simulink model "Vehicle_Model_14DOF"  (R2020a)
settings: Solver=ode23s  StartTime=0.0  StopTime=8  RelTol=1e-2  EnableMultiTasking=on
model workspace (MAT data in the model file):
  Csfl = 100
  Csfr = 100
  Csrl = 100
  Csrr = 100
  Hp = 0.35
  Ksfl = 100
  Ksfr = 100
  Ksrl = 100
  Ksrr = 100
undefined symbols (not defined in the file): sigbuilder_block
libraries: simulink_extras x6, simulink x1
(part 2 of 3)

== system Vehicle_Model_14DOF/Full vehicle 14 D.O.F /Vehicle Handling model 7D.O.F /Lateral Axis D.o.f  ==
  "ackerman outer " : Inport
  "ackerman in " : Inport  Port=2
  Fyfl : Inport  Port=3
  Fyrr : Inport  Port=4
  Fxfl : Inport  Port=5
  Fxfr : Inport  Port=6
  Fyfr : Inport  Port=7
  Fyrl : Inport  Port=8
  Vx : Inport  Port=9
  "Yaw rate " : Inport  Port=10
  "Centripital force deduction ay " : MATLAB Function  TreatAsAtomicUnit=on
  Gain : Gain  Gain=1/Ms
  Integrator : Integrator
  Integrator2 : Integrator
  MATLAB Function : MATLAB Function  TreatAsAtomicUnit=on
  Scope : Scope  NumInputPorts=2
  Scope1 : Scope
  product : Product  Inputs=**
  Y : Outport  VectorParamsAs1DForOutWhenUnconnected=off
  ay : Outport  Port=2  VectorParamsAs1DForOutWhenUnconnected=off
  Vy : Outport  Port=3  VectorParamsAs1DForOutWhenUnconnected=off
  Ay load transfer : Outport  Port=4
  wires:
  MATLAB Function/1(AY) -> Scope1/1, Gain/1  "Sprung accelration"
  Integrator2/1 -> Y/1
  Integrator/1 -> Integrator2/1, Vy/1
  "Centripital force deduction ay "/1(ay) -> ay/1, Integrator/1
  Gain/1 -> Ay load transfer/1, Scope/1, "Centripital force deduction ay "/1(Vy_dot)  "Ay"
  Vx/1 -> product/2, "Centripital force deduction ay "/2(Vx)
  "Yaw rate "/1 -> product/1, "Centripital force deduction ay "/3(Yr)
  "ackerman outer "/1 -> MATLAB Function/1(A_o)
  Fyfl/1 -> MATLAB Function/3(Fyfl)
  Fxfl/1 -> MATLAB Function/4(Fxfl)
  Fyfr/1 -> MATLAB Function/5(Fyfr)
  Fxfr/1 -> MATLAB Function/6(Fxfr)
  Fyrl/1 -> MATLAB Function/7(Fyrl)
  Fyrr/1 -> MATLAB Function/8(Fyrr)
  "ackerman in "/1 -> MATLAB Function/2(A_i)
  product/1 -> Scope/2  "V R"

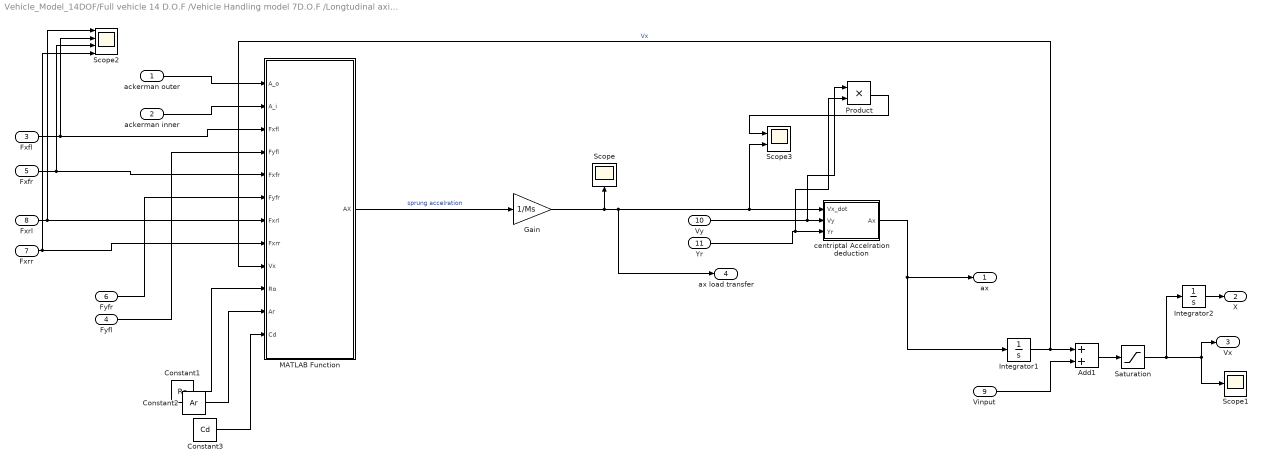
== system Vehicle_Model_14DOF/Full vehicle 14 D.O.F /Vehicle Handling model 7D.O.F /Longtudinal axis D.O.F  ==
  ackerman outer : Inport
  ackerman inner : Inport  Port=2
  Fxfl : Inport  Port=3
  Fyfl : Inport  Port=4
  Fxfr : Inport  Port=5
  Fyfr : Inport  Port=6
  Fxrr : Inport  Port=7
  Fxrl : Inport  Port=8
  Vinput : Inport  Port=9
  "Vy " : Inport  Port=10
  "Yr " : Inport  Port=11
  Add1 : Sum
  Constant1 : Constant  Value=Ro
  Constant2 : Constant  Value=Ar
  Constant3 : Constant  Value=Cd
  Gain : Gain  Gain=1/Ms
  Integrator1 : Integrator
  Integrator2 : Integrator
  MATLAB Function : MATLAB Function  TreatAsAtomicUnit=on
  Product : Product
  Saturation : Saturate  UpperLimit=inf  LowerLimit=0
  Scope : Scope
  Scope1 : Scope
  Scope2 : Scope  NumInputPorts=4
  Scope3 : Scope  NumInputPorts=2
  "centriptal Accelration deduction " : MATLAB Function  TreatAsAtomicUnit=on
  "ax " : Outport  VectorParamsAs1DForOutWhenUnconnected=off
  X : Outport  Port=2  VectorParamsAs1DForOutWhenUnconnected=off
  Vx : Outport  Port=3  VectorParamsAs1DForOutWhenUnconnected=off
  ax load transfer : Outport  Port=4
  wires:
  MATLAB Function/1(AX) -> Gain/1  "sprung accelration"
  Add1/1 -> Saturation/1
  Integrator2/1 -> X/1
  Gain/1 -> ax load transfer/1, "centriptal Accelration deduction "/1(Vx_dot), Scope3/2, Scope/1
  Vinput/1 -> Add1/2
  "centriptal Accelration deduction "/1(Ax) -> Integrator1/1, "ax "/1
  Integrator1/1 -> MATLAB Function/9(Vx), Add1/1  "Vx"
  "Yr "/1 -> Product/2, "centriptal Accelration deduction "/3(Yr)
  "Vy "/1 -> Product/1, "centriptal Accelration deduction "/2(Vy)
  ackerman outer/1 -> MATLAB Function/1(A_o)
  Fxfl/1 -> Scope2/2, MATLAB Function/3(Fxfl)
  Fyfl/1 -> MATLAB Function/4(Fyfl)
  Fxfr/1 -> Scope2/3, MATLAB Function/5(Fxfr)
  Fyfr/1 -> MATLAB Function/6(Fyfr)
  Fxrl/1 -> Scope2/1, MATLAB Function/7(Fxrl)
  Fxrr/1 -> Scope2/4, MATLAB Function/8(Fxrr)
  ackerman inner/1 -> MATLAB Function/2(A_i)
  Constant1/1 -> MATLAB Function/10(Ro)
  Constant2/1 -> MATLAB Function/11(Ar)
  Constant3/1 -> MATLAB Function/12(Cd)
  Saturation/1 -> Integrator2/1, Vx/1, Scope1/1
  Product/1 -> Scope3/1

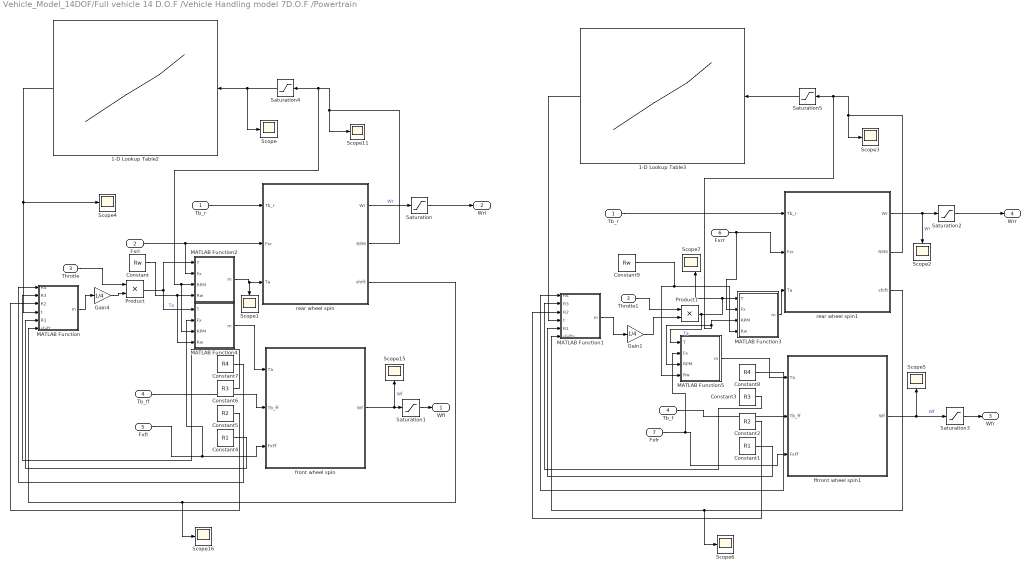
== system Vehicle_Model_14DOF/Full vehicle 14 D.O.F /Vehicle Handling model 7D.O.F /Powertrain  ==
  Tb_r : Inport
  Fxrl : Inport  Port=2
  Throtle : Inport  Port=3
  Tb_ff : Inport  Port=4
  "Fxfl " : Inport  Port=5
  Fxrr : Inport  Port=6
  Fxfr : Inport  Port=7
  1-D Lookup Table2 : Lookup_n-D  NumberOfTableDimensions=1  BreakpointsForDimension1=|  BreakpointsForDimension1FirstPoint=0  BreakpointsForDimension1Spacing=10000  Table=|  InternalRulePriority=Speed  RndMeth=Simplest  InputSameDT=on
      BreakpointsForDimension1=|
      | [ 999.991
      | 1500
      | 2000
      | 2500
      | 3000
      | 3500.01
      | 4000.02
      | 4500.01
      | 5000
      | 5500
      | 5999.99
      | 6500
      | 7000
      | 7500
      | 7999.99
      | 8499.99
      | 9000
      | 9500
      | 10000
      |   ]
      Table=|
      | [ 19.6089
      | 22.3386
      | 29.0552
      | 34.7654
      | 35.9299
      | 38.8977
      | 40.7484
      | 40.3784
      | 39.5416
      | 37.9236
      | 36.7992
      |  35.555
      | 
      | 34.3787
      | 33.134
      | 32.6401
      | 31.4746
      | 30.2131
      | 29.2355
      | 28.2404
      | ]
  1-D Lookup Table3 : Lookup_n-D  NumberOfTableDimensions=1  BreakpointsForDimension1=|  BreakpointsForDimension1FirstPoint=0  BreakpointsForDimension1Spacing=10000  Table=|  InternalRulePriority=Speed  RndMeth=Simplest  InputSameDT=on
      BreakpointsForDimension1=|
      | [ 999.991
      | 1500
      | 2000
      | 2500
      | 3000
      | 3500.01
      | 4000.02
      | 4500.01
      | 5000
      | 5500
      | 5999.99
      | 6500
      | 7000
      | 7500
      | 7999.99
      | 8499.99
      | 9000
      | 9500
      | 10000
      |   ]
      Table=|
      | [ 19.6089
      | 22.3386
      | 29.0552
      | 34.7654
      | 35.9299
      | 38.8977
      | 40.7484
      | 40.3784
      | 39.5416
      | 37.9236
      | 36.7992
      |  35.555
      | 
      | 34.3787
      | 33.134
      | 32.6401
      | 31.4746
      | 30.2131
      | 29.2355
      | 28.2404
      | ]
  Constant : Constant  Value=Rw
  Constant1 : Constant  Value=R1
  Constant2 : Constant  Value=R2
  Constant3 : Constant  Value=R3
  Constant4 : Constant  Value=R1
  Constant5 : Constant  Value=R2
  Constant6 : Constant  Value=R3
  Constant7 : Constant  Value=R4
  Constant8 : Constant  Value=R4
  Constant9 : Constant  Value=Rw
  Gain1 : Gain  Gain=1/4
  Gain4 : Gain  Gain=1/4
  MATLAB Function : MATLAB Function  TreatAsAtomicUnit=on
  MATLAB Function1 : MATLAB Function  TreatAsAtomicUnit=on
  MATLAB Function2 : MATLAB Function  TreatAsAtomicUnit=on
  MATLAB Function3 : MATLAB Function  TreatAsAtomicUnit=on
  MATLAB Function4 : MATLAB Function  TreatAsAtomicUnit=on
  MATLAB Function5 : MATLAB Function  TreatAsAtomicUnit=on
  Product : Product
  Product1 : Product
  Saturation{,1..3} (4 alike) : Saturate  UpperLimit=inf  LowerLimit=0.3745318
  Saturation4 : Saturate  UpperLimit=15000  LowerLimit=0
  Saturation5 : Saturate  UpperLimit=15000  LowerLimit=0
  Scope{,1..6,11,15..16} (10 alike) : Scope
  Scope7 : Scope  NumInputPorts=2
  "Tb_f " : InportShadow  Port=4
  "Tb_r " : InportShadow
  Throtle1 : InportShadow  Port=3
  ffrront wheel spin1 : Subsystem
  front wheel spin : Subsystem
  rear wheel spin : Subsystem
  rear wheel spin1 : Subsystem
  Wfl : Outport  VectorParamsAs1DForOutWhenUnconnected=off
  Wrl : Outport  Port=2  VectorParamsAs1DForOutWhenUnconnected=off
  Wfr : Outport  Port=3  VectorParamsAs1DForOutWhenUnconnected=off
  Wrr : Outport  Port=4  VectorParamsAs1DForOutWhenUnconnected=off
  wires:
  Fxrl/1 -> rear wheel spin/2(Fxr), MATLAB Function2/2(Fx)
  "Fxfl "/1 -> MATLAB Function4/2(Fx), front wheel spin/3(FxFf)
  1-D Lookup Table2/1 -> Scope4/1, MATLAB Function/4(t)
  rear wheel spin/2(RPM) -> MATLAB Function4/3(RPM), MATLAB Function2/3(RPM), Saturation4/1, Scope11/1
  MATLAB Function/1(m) -> Gain4/1
  rear wheel spin/1("Wr ") -> Saturation/1  "Wr"
  Tb_r/1 -> rear wheel spin/1(Tb_r)
  front wheel spin/1(Wf) -> Scope15/1, Saturation1/1  "Wf"
  Tb_ff/1 -> front wheel spin/2(Tb_ff)
  Gain4/1 -> Product/2
  rear wheel spin/3(shift) -> Scope16/1, MATLAB Function/6(shift)
  Constant4/1 -> MATLAB Function/5(R1)
  Constant5/1 -> MATLAB Function/3(R2)
  Throtle/1 -> Product/1
  Constant7/1 -> MATLAB Function/1(R4)
  Constant6/1 -> MATLAB Function/2(R3)
  Fxrr/1 -> MATLAB Function3/2(Fx), rear wheel spin1/2(Fxr)
  Fxfr/1 -> MATLAB Function5/2(Fx), ffrront wheel spin1/3(FxFf)
  1-D Lookup Table3/1 -> MATLAB Function1/4(t)
  rear wheel spin1/2(RPM) -> MATLAB Function5/3(RPM), MATLAB Function3/3(RPM), Saturation5/1, Scope3/1
  MATLAB Function1/1(m) -> Gain1/1
  rear wheel spin1/1("Wr ") -> Scope2/1, Saturation2/1  "Wr"
  Product1/1 -> MATLAB Function5/1(T), Scope7/2, MATLAB Function3/1(T)  "Ta"
  "Tb_r "/1 -> rear wheel spin1/1(Tb_r)
  ffrront wheel spin1/1(Wf) -> Scope5/1, Saturation3/1  "Wf"
  "Tb_f "/1 -> ffrront wheel spin1/2(Tb_ff)
  Gain1/1 -> Product1/2
  rear wheel spin1/3(shift) -> MATLAB Function1/6(shifts), Scope6/1
  Constant1/1 -> MATLAB Function1/5(R1)
  Constant2/1 -> MATLAB Function1/3(R2)
  Constant8/1 -> MATLAB Function1/1(R4)
  Constant3/1 -> MATLAB Function1/2(R3)
  Throtle1/1 -> Product1/1
  Saturation/1 -> Wrl/1
  Saturation1/1 -> Wfl/1
  Saturation2/1 -> Wrr/1
  Saturation3/1 -> Wfr/1
  Saturation4/1 -> 1-D Lookup Table2/1, Scope/1
  Saturation5/1 -> 1-D Lookup Table3/1
  Product/1 -> MATLAB Function4/1(T), MATLAB Function2/1(T)  "Ta"
  MATLAB Function2/1(m) -> Scope1/1, rear wheel spin/3(Ta)
  MATLAB Function3/1(m) -> rear wheel spin1/3(Ta)
  MATLAB Function4/1(m) -> front wheel spin/1(Ta)
  MATLAB Function5/1(m) -> ffrront wheel spin1/1(Ta)
  Constant/1 -> MATLAB Function4/4(Rw), MATLAB Function2/4(Rw)
  Constant9/1 -> MATLAB Function3/4(Rw), MATLAB Function5/4(Rw)

== system Vehicle_Model_14DOF/Full vehicle 14 D.O.F /Vehicle Handling model 7D.O.F /Slip angle and beta  ==
  ackerman angle outer : Inport
  "ackerman angle Inner " : Inport  Port=2
  Yaw rate : Inport  Port=3
  Vx : Inport  Port=4
  "Vy  " : Inport  Port=5
  Slip angle front : Subsystem
  Slip angle front1 : Subsystem
  Slip angle rear : Subsystem
  Slip angle rear1 : Subsystem
  "Vx  " : InportShadow  Port=4
  "Vx        " : InportShadow  Port=4
  "Vx         " : InportShadow  Port=4
  "Vy     " : InportShadow  Port=5
  "Vy        " : InportShadow  Port=5
  "Vy         " : InportShadow  Port=5
  "Yaw rate      " : InportShadow  Port=3
  "Yaw rate         " : InportShadow  Port=3
  "Yaw rate          " : InportShadow  Port=3
  alpha_fl : Outport  VectorParamsAs1DForOutWhenUnconnected=off
  alpha_fr : Outport  Port=2  VectorParamsAs1DForOutWhenUnconnected=off
  alpha_rl : Outport  Port=3  VectorParamsAs1DForOutWhenUnconnected=off
  alpha_rr : Outport  Port=4  VectorParamsAs1DForOutWhenUnconnected=off
  wires:
  Slip angle rear/1(alpha_R) -> alpha_rl/1  "rl"
  Slip angle front1/1(alpha_F) -> alpha_fr/1  "fl"
  Slip angle rear1/1(alpha_R) -> alpha_rr/1  "rl"
  ackerman angle outer/1 -> Slip angle front/2(Delta)
  "Vy     "/1 -> Slip angle front/3(Ydot)
  Yaw rate/1 -> Slip angle front/4(Psidot)
  Vx/1 -> Slip angle front/1(Xdot)
  "Vx        "/1 -> Slip angle front1/1(Xdot)
  "Yaw rate         "/1 -> Slip angle front1/4(Psidot)
  "Vy        "/1 -> Slip angle front1/3(Ydot)
  "ackerman angle Inner "/1 -> Slip angle front1/2(Delta)
  Slip angle front/1(alpha_F) -> alpha_fl/1  "fl"
  "Vy         "/1 -> Slip angle rear1/2(Ydot)
  "Yaw rate          "/1 -> Slip angle rear1/3(Psidot)
  "Vx         "/1 -> Slip angle rear1/1(Xdot)
  "Vy  "/1 -> Slip angle rear/2(Ydot)
  "Vx  "/1 -> Slip angle rear/1(Xdot)
  "Yaw rate      "/1 -> Slip angle rear/3(Psidot)

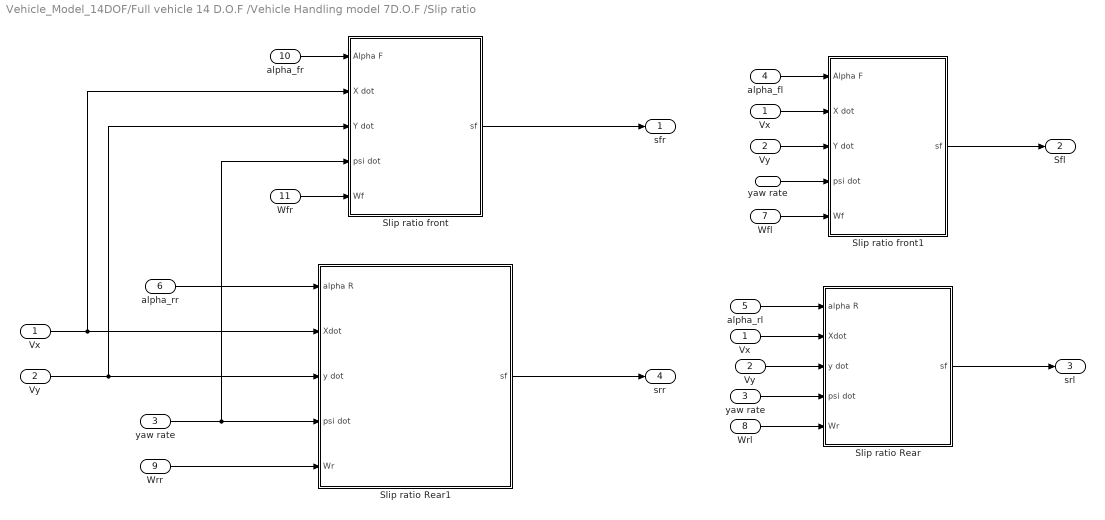
== system Vehicle_Model_14DOF/Full vehicle 14 D.O.F /Vehicle Handling model 7D.O.F /Slip ratio  ==
  "Vx " : Inport
  Vy : Inport  Port=2
  yaw rate : Inport  Port=3
  alpha_fl : Inport  Port=4
  "alpha_rl " : Inport  Port=5
  alpha_rr : Inport  Port=6
  "Wfl " : Inport  Port=7
  Wrl : Inport  Port=8
  Wrr : Inport  Port=9
  alpha_fr : Inport  Port=10
  Wfr : Inport  Port=11
  Slip ratio Rear : Subsystem
  Slip ratio Rear1 : Subsystem
  Slip ratio front : Subsystem
  Slip ratio front1 : Subsystem
  "Vx " : InportShadow
  "Vx " : InportShadow
  "Vy " : InportShadow  Port=2
  "Vy " : InportShadow  Port=2
  "yaw rate " : InportShadow  Port=3
  "yaw rate        " : InportShadow  Port=3
  sfr : Outport  VectorParamsAs1DForOutWhenUnconnected=off
  Sfl : Outport  Port=2  VectorParamsAs1DForOutWhenUnconnected=off
  srl : Outport  Port=3  VectorParamsAs1DForOutWhenUnconnected=off
  srr : Outport  Port=4  VectorParamsAs1DForOutWhenUnconnected=off
  wires:
  "yaw rate        "/1 -> Slip ratio front/4(psi dot), Slip ratio Rear1/4(psi dot)
  alpha_rr/1 -> Slip ratio Rear1/1(alpha R)
  "Vx "/1 -> Slip ratio front1/2(X dot)
  Vy/1 -> Slip ratio front1/3(Y dot)
  yaw rate/1 -> Slip ratio front1/4(psi dot)
  alpha_fl/1 -> Slip ratio front1/1(Alpha F)
  "Vx "/1 -> Slip ratio Rear/2(Xdot)
  "Vy "/1 -> Slip ratio Rear/3(y dot)
  "yaw rate "/1 -> Slip ratio Rear/4(psi dot)
  "alpha_rl "/1 -> Slip ratio Rear/1(alpha R)
  Wrr/1 -> Slip ratio Rear1/5(Wr)
  Wrl/1 -> Slip ratio Rear/5(Wr)
  "Wfl "/1 -> Slip ratio front1/5(Wf)
  Slip ratio Rear1/1(sf) -> srr/1
  Slip ratio front1/1(sf) -> Sfl/1
  Slip ratio Rear/1(sf) -> srl/1
  Slip ratio front/1(sf) -> sfr/1
  Wfr/1 -> Slip ratio front/5(Wf)
  alpha_fr/1 -> Slip ratio front/1(Alpha F)
  "Vy "/1 -> Slip ratio front/3(Y dot), Slip ratio Rear1/3(y dot)
  "Vx "/1 -> Slip ratio front/2(X dot), Slip ratio Rear1/2(Xdot)

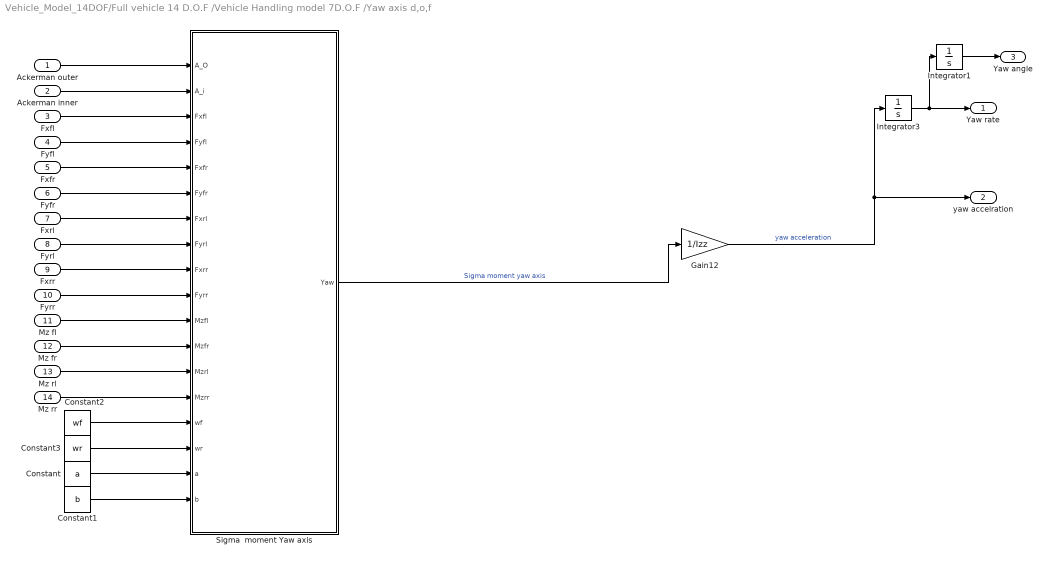
== system Vehicle_Model_14DOF/Full vehicle 14 D.O.F /Vehicle Handling model 7D.O.F /Yaw axis d,o,f  ==
  "Ackerman outer " : Inport
  "Ackerman inner " : Inport  Port=2
  Fxfl : Inport  Port=3
  "Fyfl " : Inport  Port=4
  Fxfr : Inport  Port=5
  Fyfr : Inport  Port=6
  Fxrl : Inport  Port=7
  Fyrl : Inport  Port=8
  Fxrr : Inport  Port=9
  Fyrr : Inport  Port=10
  Mz fl : Inport  Port=11
  Mz fr : Inport  Port=12
  Mz rl : Inport  Port=13
  Mz rr : Inport  Port=14
  Constant : Constant  Value=a
  Constant1 : Constant  Value=b
  Constant2 : Constant  Value=wf
  Constant3 : Constant  Value=wr
  Gain12 : Gain  Gain=1/Izz
  Integrator1 : Integrator  ZeroCross=off
  Integrator3 : Integrator  ZeroCross=off
  Sigma  moment Yaw axis : MATLAB Function  TreatAsAtomicUnit=on
  "Yaw rate " : Outport  VectorParamsAs1DForOutWhenUnconnected=off
  "yaw accelration " : Outport  Port=2  VectorParamsAs1DForOutWhenUnconnected=off
  Yaw angle : Outport  Port=3  VectorParamsAs1DForOutWhenUnconnected=off
  wires:
  Sigma  moment Yaw axis/1(Yaw) -> Gain12/1  "Sigma moment yaw axis"
  Integrator3/1 -> Integrator1/1, "Yaw rate "/1
  Gain12/1 -> Integrator3/1, "yaw accelration "/1  "yaw acceleration"
  Integrator1/1 -> Yaw angle/1
  "Ackerman outer "/1 -> Sigma  moment Yaw axis/1(A_O)
  Fxfl/1 -> Sigma  moment Yaw axis/3(Fxfl)
  "Fyfl "/1 -> Sigma  moment Yaw axis/4(Fyfl)
  Fxfr/1 -> Sigma  moment Yaw axis/5(Fxfr)
  Fyfr/1 -> Sigma  moment Yaw axis/6(Fyfr)
  Fxrl/1 -> Sigma  moment Yaw axis/7(Fxrl)
  Fyrl/1 -> Sigma  moment Yaw axis/8(Fyrl)
  Fxrr/1 -> Sigma  moment Yaw axis/9(Fxrr)
  Fyrr/1 -> Sigma  moment Yaw axis/10(Fyrr)
  Mz fl/1 -> Sigma  moment Yaw axis/11(Mzfl)
  Mz fr/1 -> Sigma  moment Yaw axis/12(Mzfr)
  Mz rl/1 -> Sigma  moment Yaw axis/13(Mzrl)
  Mz rr/1 -> Sigma  moment Yaw axis/14(Mzrr)
  Constant/1 -> Sigma  moment Yaw axis/17(a)
  Constant1/1 -> Sigma  moment Yaw axis/18(b)
  Constant2/1 -> Sigma  moment Yaw axis/15(wf)
  Constant3/1 -> Sigma  moment Yaw axis/16(wr)
  "Ackerman inner "/1 -> Sigma  moment Yaw axis/2(A_i)

== system Vehicle_Model_14DOF/Full vehicle 14 D.O.F /RIde1/Subsys Fz/Subsys Fzfl ==
  note: mufl.g
  note: Ms.g
  note: Ms.gb
  note: a+b
  note: 2(a+b)
  note: Msg.b/2(a+b)
  Ffl : Inport
  Downforce : Inport  Port=2
  Add : Sum
  Add1 : Sum  Inputs=++++
  Divide : Product  Inputs=*/
  Ms : Constant  Value=Ms
  Product3 : Product  RndMeth=Zero
  a : Constant  Value=a
  b : Constant  Value=b
  constant : Gain  Gain=2
  g : Gain  Gain=9.81
  g1 : Gain  Gain=9.81
  mufl : Constant  Value=Mufl
  Fzfl : Outport  VectorParamsAs1DForOutWhenUnconnected=off
  wires:
  b/1 -> Add/1, Product3/2
  Product3/1 -> Divide/1
  a/1 -> Add/2
  Add/1 -> constant/1
  constant/1 -> Divide/2
  mufl/1 -> g/1
  g/1 -> Add1/2
  Ms/1 -> g1/1
  g1/1 -> Product3/1
  Divide/1 -> Add1/1
  Ffl/1 -> Add1/3
  Add1/1 -> Fzfl/1
  Downforce/1 -> Add1/4

== system Vehicle_Model_14DOF/Full vehicle 14 D.O.F /RIde1/Subsys Fz/Subsys Fzfr ==
  note: Msg.b/2(a+b)
  note: 2(a+b)
  note: a+b
  note: Ms.gb
  note: Ms.g
  note: mufr.g
  Ffr : Inport
  Downforce : Inport  Port=2
  Add : Sum
  Add1 : Sum  Inputs=++++
  Divide : Product  Inputs=*/
  Ms : Constant  Value=Ms
  Product3 : Product  RndMeth=Zero
  a : Constant  Value=a
  b : Constant  Value=b
  constant : Gain  Gain=2
  g : Gain  Gain=9.81
  g1 : Gain  Gain=9.81
  mufr : Constant  Value=Mufr
  Fzfr : Outport  VectorParamsAs1DForOutWhenUnconnected=off
  wires:
  Add1/1 -> Fzfr/1
  Ffr/1 -> Add1/3
  Divide/1 -> Add1/1
  g1/1 -> Product3/1
  Ms/1 -> g1/1
  g/1 -> Add1/2
  mufr/1 -> g/1
  constant/1 -> Divide/2
  Add/1 -> constant/1
  a/1 -> Add/2
  Product3/1 -> Divide/1
  b/1 -> Add/1, Product3/2
  Downforce/1 -> Add1/4

== system Vehicle_Model_14DOF/Full vehicle 14 D.O.F /RIde1/Subsys Fz/Subsys Fzrl ==
  note: Msg.a/2(a+b)
  note: 2(a+b)
  note: a+b
  note: Ms.ga
  note: Ms.g
  note: murl.g
  Frl : Inport
  downforce : Inport  Port=2
  Add : Sum
  Add1 : Sum  Inputs=++++
  Divide : Product  Inputs=*/
  Ms : Constant  Value=Ms
  Product3 : Product  RndMeth=Zero
  a : Constant  Value=a
  b : Constant  Value=b
  constant : Gain  Gain=2
  g : Gain  Gain=9.81
  g1 : Gain  Gain=9.81
  mufl : Constant  Value=Murl
  Fzrl : Outport  VectorParamsAs1DForOutWhenUnconnected=off
  wires:
  Add1/1 -> Fzrl/1
  Frl/1 -> Add1/3
  Divide/1 -> Add1/1
  g1/1 -> Product3/1
  Ms/1 -> g1/1
  g/1 -> Add1/2
  mufl/1 -> g/1
  constant/1 -> Divide/2
  Add/1 -> constant/1
  b/1 -> Add/2
  Product3/1 -> Divide/1
  a/1 -> Add/1, Product3/2
  downforce/1 -> Add1/4

== system Vehicle_Model_14DOF/Full vehicle 14 D.O.F /RIde1/Subsys Fz/Subsys Fzrl1 ==
  note: murr.g
  note: Ms.g
  note: Ms.ga
  note: a+b
  note: 2(a+b)
  note: Msg.a/2(a+b)
  Frr : Inport
  downforce : Inport  Port=2
  Add : Sum
  Add1 : Sum  Inputs=++++
  Divide : Product  Inputs=*/
  Ms : Constant  Value=Ms
  Product3 : Product  RndMeth=Zero
  a : Constant  Value=a
  b : Constant  Value=b
  constant : Gain  Gain=2
  g : Gain  Gain=9.81
  g1 : Gain  Gain=9.81
  murr : Constant  Value=Murr
  Fzrr : Outport  VectorParamsAs1DForOutWhenUnconnected=off
  wires:
  a/1 -> Product3/2, Add/1
  Product3/1 -> Divide/1
  b/1 -> Add/2
  Add/1 -> constant/1
  constant/1 -> Divide/2
  murr/1 -> g/1
  g/1 -> Add1/2
  Ms/1 -> g1/1
  g1/1 -> Product3/1
  Divide/1 -> Add1/1
  Frr/1 -> Add1/3
  Add1/1 -> Fzrr/1
  downforce/1 -> Add1/4

== system Vehicle_Model_14DOF/Full vehicle 14 D.O.F /Tiremodel/LCO width 6 psi 10/Fx ==
  Fz : Inport
  In3 : Inport  Port=2
  MATLAB Function : MATLAB Function  TreatAsAtomicUnit=on
  "Fx  " : Outport  VectorParamsAs1DForOutWhenUnconnected=off
  wires:
  Fz/1 -> MATLAB Function/1(ffz)
  In3/1 -> MATLAB Function/2(xx)
  MATLAB Function/1(Fx) -> "Fx  "/1

== system Vehicle_Model_14DOF/Full vehicle 14 D.O.F /Tiremodel/LCO width 6 psi 10/fy ==
  Fz : Inport
  Slip angle : Inport  Port=2
  MATLAB Function : MATLAB Function  TreatAsAtomicUnit=on
  "Fy  " : Outport  VectorParamsAs1DForOutWhenUnconnected=off
  wires:
  Fz/1 -> MATLAB Function/1(ffz)
  Slip angle/1 -> MATLAB Function/2(xx)
  MATLAB Function/1(Fx) -> "Fy  "/1

== system Vehicle_Model_14DOF/Full vehicle 14 D.O.F /Tiremodel/LCO width 6 psi 10/fy1 ==
  Fz1 : Inport
  alpha : Inport  Port=2
  MZ : Subsystem
  mmz : Outport  VectorParamsAs1DForOutWhenUnconnected=off
  wires:
  MZ/1(MZ) -> mmz/1
  Fz1/1 -> MZ/1(Fz)
  alpha/1 -> MZ/2(Slip angle)

== system Vehicle_Model_14DOF/Full vehicle 14 D.O.F /Tiremodel/LCO width 6 psi 14/Fx ==
  Fz : Inport
  In3 : Inport  Port=2
  MATLAB Function : MATLAB Function  TreatAsAtomicUnit=on
  "Fx  " : Outport  VectorParamsAs1DForOutWhenUnconnected=off
  wires:
  Fz/1 -> MATLAB Function/1(ffz)
  In3/1 -> MATLAB Function/2(xx)
  MATLAB Function/1(Fx) -> "Fx  "/1

== system Vehicle_Model_14DOF/Full vehicle 14 D.O.F /Tiremodel/LCO width 6 psi 14/fy ==
  Fz : Inport
  Slip angle : Inport  Port=2
  MATLAB Function : MATLAB Function  TreatAsAtomicUnit=on
  "Fy  " : Outport  VectorParamsAs1DForOutWhenUnconnected=off
  wires:
  Fz/1 -> MATLAB Function/1(ffz)
  Slip angle/1 -> MATLAB Function/2(xx)
  MATLAB Function/1(Fx) -> "Fy  "/1

== system Vehicle_Model_14DOF/Full vehicle 14 D.O.F /Tiremodel/LCO width 6 psi 14/fy1 ==
  Fz1 : Inport
  alpha : Inport  Port=2
  MZ : Subsystem
  mmz : Outport  VectorParamsAs1DForOutWhenUnconnected=off
  wires:
  MZ/1(MZ) -> mmz/1
  Fz1/1 -> MZ/1(Fz)
  alpha/1 -> MZ/2(Slip angle)

== system Vehicle_Model_14DOF/Full vehicle 14 D.O.F /Tiremodel/R25b width 6 psi 10/Fx ==
  Fz : Inport
  In3 : Inport  Port=2
  MATLAB Function : MATLAB Function  TreatAsAtomicUnit=on
  "Fx  " : Outport  VectorParamsAs1DForOutWhenUnconnected=off
  wires:
  Fz/1 -> MATLAB Function/1(ffz)
  In3/1 -> MATLAB Function/2(xx)
  MATLAB Function/1(Fx) -> "Fx  "/1

== system Vehicle_Model_14DOF/Full vehicle 14 D.O.F /Tiremodel/R25b width 6 psi 10/fy ==
  Fz : Inport
  Slip angle : Inport  Port=2
  MATLAB Function : MATLAB Function  TreatAsAtomicUnit=on
  "Fy  " : Outport  VectorParamsAs1DForOutWhenUnconnected=off
  wires:
  Fz/1 -> MATLAB Function/1(ffz)
  Slip angle/1 -> MATLAB Function/2(xx)
  MATLAB Function/1(Fx) -> "Fy  "/1

== system Vehicle_Model_14DOF/Full vehicle 14 D.O.F /Tiremodel/R25b width 6 psi 10/fy1 ==
  Fz1 : Inport
  alpha : Inport  Port=2
  MZ : Subsystem
  mmz : Outport  VectorParamsAs1DForOutWhenUnconnected=off
  wires:
  MZ/1(MZ) -> mmz/1
  Fz1/1 -> MZ/1(Fz)
  alpha/1 -> MZ/2(Slip angle)

== system Vehicle_Model_14DOF/Full vehicle 14 D.O.F /Tiremodel/R25b width 6 psi 14/Fx ==
  Fz : Inport
  In3 : Inport  Port=2
  MATLAB Function : MATLAB Function  TreatAsAtomicUnit=on
  "Fx  " : Outport  VectorParamsAs1DForOutWhenUnconnected=off
  wires:
  Fz/1 -> MATLAB Function/1(ffz)
  In3/1 -> MATLAB Function/2(xx)
  MATLAB Function/1(Fx) -> "Fx  "/1

== system Vehicle_Model_14DOF/Full vehicle 14 D.O.F /Tiremodel/R25b width 6 psi 14/fy ==
  Fz : Inport
  Slip angle : Inport  Port=2
  MATLAB Function : MATLAB Function  TreatAsAtomicUnit=on
  "Fy  " : Outport  VectorParamsAs1DForOutWhenUnconnected=off
  wires:
  Fz/1 -> MATLAB Function/1(ffz)
  Slip angle/1 -> MATLAB Function/2(xx)
  MATLAB Function/1(Fx) -> "Fy  "/1

== system Vehicle_Model_14DOF/Full vehicle 14 D.O.F /Tiremodel/R25b width 6 psi 14/fy1 ==
  Fz1 : Inport
  alpha : Inport  Port=2
  MZ : Subsystem
  mmz : Outport  VectorParamsAs1DForOutWhenUnconnected=off
  wires:
  MZ/1(MZ) -> mmz/1
  Fz1/1 -> MZ/1(Fz)
  alpha/1 -> MZ/2(Slip angle)

== system Vehicle_Model_14DOF/Full vehicle 14 D.O.F /Tiremodel/R25b width 7 psi 10/Fx ==
  Fz : Inport
  In3 : Inport  Port=2
  MATLAB Function : MATLAB Function  TreatAsAtomicUnit=on
  "Fx  " : Outport  VectorParamsAs1DForOutWhenUnconnected=off
  wires:
  Fz/1 -> MATLAB Function/1(ffz)
  In3/1 -> MATLAB Function/2(xx)
  MATLAB Function/1(Fx) -> "Fx  "/1

== system Vehicle_Model_14DOF/Full vehicle 14 D.O.F /Tiremodel/R25b width 7 psi 10/MZ ==
  Fz1 : Inport
  alpha : Inport  Port=2
  MZ : Subsystem
  mmz : Outport  VectorParamsAs1DForOutWhenUnconnected=off
  wires:
  MZ/1(MZ) -> mmz/1
  Fz1/1 -> MZ/1(Fz)
  alpha/1 -> MZ/2(Slip angle)

== system Vehicle_Model_14DOF/Full vehicle 14 D.O.F /Tiremodel/R25b width 7 psi 10/fy ==
  Fz : Inport
  Slip angle : Inport  Port=2
  MATLAB Function : MATLAB Function  TreatAsAtomicUnit=on
  "Fy  " : Outport  VectorParamsAs1DForOutWhenUnconnected=off
  wires:
  Fz/1 -> MATLAB Function/1(ffz)
  Slip angle/1 -> MATLAB Function/2(xx)
  MATLAB Function/1(Fx) -> "Fy  "/1

== system Vehicle_Model_14DOF/Full vehicle 14 D.O.F /Tiremodel/R25b width 7 psi 14/Fx ==
  Fz : Inport
  In3 : Inport  Port=2
  MATLAB Function : MATLAB Function  TreatAsAtomicUnit=on
  "Fx  " : Outport  VectorParamsAs1DForOutWhenUnconnected=off
  wires:
  Fz/1 -> MATLAB Function/1(ffz)
  In3/1 -> MATLAB Function/2(xx)
  MATLAB Function/1(Fx) -> "Fx  "/1

== system Vehicle_Model_14DOF/Full vehicle 14 D.O.F /Tiremodel/R25b width 7 psi 14/fy ==
  Fz : Inport
  Slip angle : Inport  Port=2
  MATLAB Function : MATLAB Function  TreatAsAtomicUnit=on
  "Fy  " : Outport  VectorParamsAs1DForOutWhenUnconnected=off
  wires:
  Fz/1 -> MATLAB Function/1(ffz)
  Slip angle/1 -> MATLAB Function/2(xx)
  MATLAB Function/1(Fx) -> "Fy  "/1

== system Vehicle_Model_14DOF/Full vehicle 14 D.O.F /Tiremodel/R25b width 7 psi 14/fy1 ==
  Fz1 : Inport
  alpha : Inport  Port=2
  MZ : Subsystem
  mmz : Outport  VectorParamsAs1DForOutWhenUnconnected=off
  wires:
  MZ/1(MZ) -> mmz/1
  Fz1/1 -> MZ/1(Fz)
  alpha/1 -> MZ/2(Slip angle)

== system Vehicle_Model_14DOF/Full vehicle 14 D.O.F /Tiremodel/Tire front left/Fx ==
  Fz : Inport
  S : Inport  Port=2
  MATLAB Function : MATLAB Function  TreatAsAtomicUnit=on
  "Fx  " : Outport  VectorParamsAs1DForOutWhenUnconnected=off
  wires:
  Fz/1 -> MATLAB Function/1(ffz)
  S/1 -> MATLAB Function/2(xx)
  MATLAB Function/1(Fx) -> "Fx  "/1

== system Vehicle_Model_14DOF/Full vehicle 14 D.O.F /Tiremodel/Tire front left/fy ==
  Fz : Inport
  Slip angle : Inport  Port=2
  MATLAB Function : MATLAB Function  TreatAsAtomicUnit=on
  "Fy  " : Outport  VectorParamsAs1DForOutWhenUnconnected=off
  wires:
  Fz/1 -> MATLAB Function/1(ffz)
  Slip angle/1 -> MATLAB Function/2(xx)
  MATLAB Function/1(Fx) -> "Fy  "/1

== system Vehicle_Model_14DOF/Full vehicle 14 D.O.F /Tiremodel/Tire front left/fy1 ==
  Fz1 : Inport
  alpha : Inport  Port=2
  MZ : Subsystem
  mmz : Outport  VectorParamsAs1DForOutWhenUnconnected=off
  wires:
  MZ/1(MZ) -> mmz/1
  Fz1/1 -> MZ/1(Fz)
  alpha/1 -> MZ/2(Slip angle)

== system Vehicle_Model_14DOF/Full vehicle 14 D.O.F /Tiremodel/Tire front right/Fx ==
  Fz : Inport
  In3 : Inport  Port=2
  MATLAB Function : MATLAB Function  TreatAsAtomicUnit=on
  "Fx  " : Outport  VectorParamsAs1DForOutWhenUnconnected=off
  wires:
  MATLAB Function/1(Fx) -> "Fx  "/1
  In3/1 -> MATLAB Function/2(xx)
  Fz/1 -> MATLAB Function/1(ffz)

== system Vehicle_Model_14DOF/Full vehicle 14 D.O.F /Tiremodel/Tire front right/fy ==
  Fz : Inport
  Slip angle : Inport  Port=2
  MATLAB Function : MATLAB Function  TreatAsAtomicUnit=on
  "Fy  " : Outport  VectorParamsAs1DForOutWhenUnconnected=off
  wires:
  MATLAB Function/1(Fx) -> "Fy  "/1
  Slip angle/1 -> MATLAB Function/2(xx)
  Fz/1 -> MATLAB Function/1(ffz)

== system Vehicle_Model_14DOF/Full vehicle 14 D.O.F /Tiremodel/Tire front right/fy1 ==
  Fz1 : Inport
  alpha : Inport  Port=2
  MZ : Subsystem
  mmz : Outport  VectorParamsAs1DForOutWhenUnconnected=off
  wires:
  alpha/1 -> MZ/2(Slip angle)
  Fz1/1 -> MZ/1(Fz)
  MZ/1(MZ) -> mmz/1

== system Vehicle_Model_14DOF/Full vehicle 14 D.O.F /Tiremodel/Tire rear Right/Fx ==
  Fz : Inport
  In3 : Inport  Port=2
  MATLAB Function : MATLAB Function  TreatAsAtomicUnit=on
  "Fx  " : Outport  VectorParamsAs1DForOutWhenUnconnected=off
  wires:
  Fz/1 -> MATLAB Function/1(ffz)
  In3/1 -> MATLAB Function/2(xx)
  MATLAB Function/1(Fx) -> "Fx  "/1

== system Vehicle_Model_14DOF/Full vehicle 14 D.O.F /Tiremodel/Tire rear Right/fy ==
  Fz : Inport
  Slip angle : Inport  Port=2
  MATLAB Function : MATLAB Function  TreatAsAtomicUnit=on
  "Fy  " : Outport  VectorParamsAs1DForOutWhenUnconnected=off
  wires:
  Fz/1 -> MATLAB Function/1(ffz)
  Slip angle/1 -> MATLAB Function/2(xx)
  MATLAB Function/1(Fx) -> "Fy  "/1

== system Vehicle_Model_14DOF/Full vehicle 14 D.O.F /Tiremodel/Tire rear Right/fy1 ==
  Fz1 : Inport
  alpha : Inport  Port=2
  MZ : Subsystem
  mmz : Outport  VectorParamsAs1DForOutWhenUnconnected=off
  wires:
  MZ/1(MZ) -> mmz/1
  Fz1/1 -> MZ/1(Fz)
  alpha/1 -> MZ/2(Slip angle)

== system Vehicle_Model_14DOF/Full vehicle 14 D.O.F /Tiremodel/Tire rear left/Fx ==
  Fz : Inport
  In3 : Inport  Port=2
  MATLAB Function : MATLAB Function  TreatAsAtomicUnit=on
  "Fx  " : Outport  VectorParamsAs1DForOutWhenUnconnected=off
  wires:
  MATLAB Function/1(Fx) -> "Fx  "/1
  In3/1 -> MATLAB Function/2(xx)
  Fz/1 -> MATLAB Function/1(ffz)

== system Vehicle_Model_14DOF/Full vehicle 14 D.O.F /Tiremodel/Tire rear left/fy ==
  Fz : Inport
  Slip angle : Inport  Port=2
  MATLAB Function : MATLAB Function  TreatAsAtomicUnit=on
  "Fy  " : Outport  VectorParamsAs1DForOutWhenUnconnected=off
  wires:
  MATLAB Function/1(Fx) -> "Fy  "/1
  Slip angle/1 -> MATLAB Function/2(xx)
  Fz/1 -> MATLAB Function/1(ffz)

== system Vehicle_Model_14DOF/Full vehicle 14 D.O.F /Tiremodel/Tire rear left/fy1 ==
  Fz1 : Inport
  alpha : Inport  Port=2
  MZ : Subsystem
  mmz : Outport  VectorParamsAs1DForOutWhenUnconnected=off
  wires:
  alpha/1 -> MZ/2(Slip angle)
  Fz1/1 -> MZ/1(Fz)
  MZ/1(MZ) -> mmz/1

== system Vehicle_Model_14DOF/Full vehicle 14 D.O.F /Vehicle Handling model 7D.O.F /Powertrain /ffrront wheel spin1 ==
  Ta : Inport
  Tb_ff : Inport  Port=2
  FxFf : Inport  Port=3
  Add : Sum  Inputs=+--
  Gain : Gain  Gain=Rw
  Gain1 : Gain  Gain=1/Iwf
  Integrator : Integrator  InitialCondition=0.1
  One : Constant  OutDataTypeStr=Inherit: Inherit via back propagation
  Product : Product
  Scope : Scope  NumInputPorts=2
  Scope1 : Scope
  Scope4 : Scope
  Sign : Signum
  Terminator : Terminator
  Wf : Outport  VectorParamsAs1DForOutWhenUnconnected=off
  wires:
  One/1 -> Product/2
  Product/1 -> Add/2, Scope/1
  Gain/1 -> Add/3, Scope/2
  Sign/1 -> Terminator/1
  Add/1 -> Gain1/1
  Tb_ff/1 -> Product/1
  Integrator/1 -> Wf/1, Scope4/1, Sign/1
  Ta/1 -> Add/1, Scope1/1
  FxFf/1 -> Gain/1
  Gain1/1 -> Integrator/1

== system Vehicle_Model_14DOF/Full vehicle 14 D.O.F /Vehicle Handling model 7D.O.F /Powertrain /front wheel spin ==
  Ta : Inport
  Tb_ff : Inport  Port=2
  FxFf : Inport  Port=3
  Add : Sum  Inputs=+--
  Gain : Gain  Gain=Rw
  Gain1 : Gain  Gain=1/Iwf
  Integrator : Integrator  InitialCondition=0.1
  One : Constant  OutDataTypeStr=Inherit: Inherit via back propagation
  Product : Product
  Scope : Scope  NumInputPorts=2
  Scope1 : Scope  NumInputPorts=2
  Scope4 : Scope
  Sign : Signum
  Terminator : Terminator
  Wf : Outport  VectorParamsAs1DForOutWhenUnconnected=off
  wires:
  Gain1/1 -> Integrator/1
  FxFf/1 -> Gain/1
  Ta/1 -> Scope1/1, Add/1
  Integrator/1 -> Scope4/1, Sign/1, Wf/1
  Tb_ff/1 -> Product/1
  Add/1 -> Gain1/1
  Sign/1 -> Terminator/1
  Gain/1 -> Scope/2, Add/3, Scope1/2
  Product/1 -> Scope/1, Add/2
  One/1 -> Product/2

== system Vehicle_Model_14DOF/Full vehicle 14 D.O.F /Vehicle Handling model 7D.O.F /Powertrain /rear wheel spin ==
  Tb_r : Inport
  Fxr : Inport  Port=2
  Ta : Inport  Port=3
  Add : Sum  Inputs=+--
  Add1 : Sum
  Constant : Constant
  Constant1 : Constant  Value=R1
  Constant2 : Constant  Value=R2
  Constant3 : Constant  Value=R3
  Constant4 : Constant  Value=R4
  Gain : Gain  Gain=Rw
  Gain1 : Gain  Gain=1/Iwf
  Integrator : Integrator  InitialCondition=0.1
  MATLAB Function : MATLAB Function  TreatAsAtomicUnit=on
  MATLAB Function1 : MATLAB Function  TreatAsAtomicUnit=on
  Memory : Memory  InitialCondition=1
  One : Constant  OutDataTypeStr=Inherit: Inherit via back propagation
  Product : Product
  Scope : Scope  NumInputPorts=2
  "Wr " : Outport  VectorParamsAs1DForOutWhenUnconnected=off
  RPM : Outport  Port=2  VectorParamsAs1DForOutWhenUnconnected=off
  shift : Outport  Port=3  VectorParamsAs1DForOutWhenUnconnected=off
  wires:
  Gain1/1 -> Integrator/1
  Gain/1 -> Scope/1, Add/2  "Fxr"
  Fxr/1 -> Gain/1
  Ta/1 -> Add/1, Scope/2  "Ta"
  Integrator/1 -> MATLAB Function/5(u)
  MATLAB Function/1(y) -> "Wr "/1
  MATLAB Function/3(shift) -> Memory/1
  Constant/1 -> Add1/1
  Add1/1 -> shift/1, MATLAB Function/6("shift ")
  MATLAB Function1/1(y) -> Add1/2
  Memory/1 -> MATLAB Function1/1(u)
  Constant4/1 -> MATLAB Function/1(R4)
  Constant3/1 -> MATLAB Function/2(R3)
  Constant2/1 -> MATLAB Function/3(R2)
  Constant1/1 -> MATLAB Function/4(R1)
  Tb_r/1 -> Product/1
  Add/1 -> Gain1/1
  Product/1 -> Add/3
  One/1 -> Product/2
  MATLAB Function/2(RPM) -> RPM/1

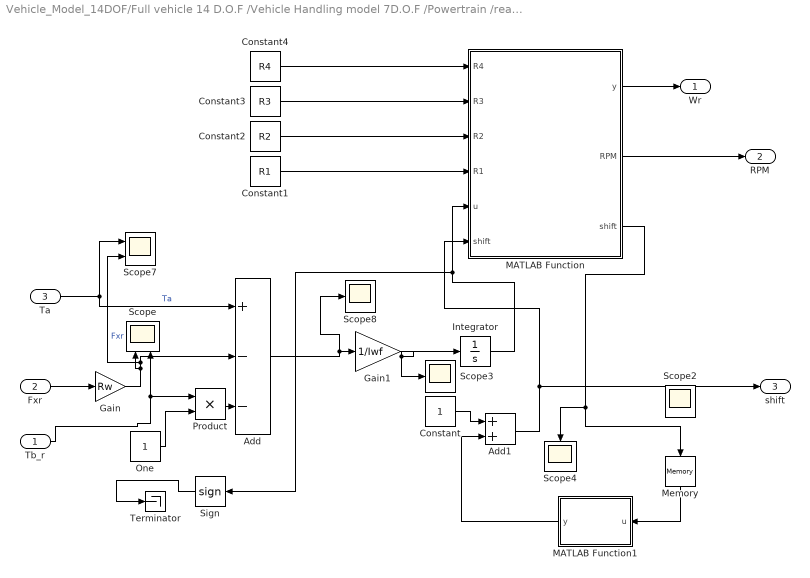
== system Vehicle_Model_14DOF/Full vehicle 14 D.O.F /Vehicle Handling model 7D.O.F /Powertrain /rear wheel spin1 ==
  Tb_r : Inport
  Fxr : Inport  Port=2
  Ta : Inport  Port=3
  Add : Sum  Inputs=+--
  Add1 : Sum
  Constant : Constant
  Constant1 : Constant  Value=R1
  Constant2 : Constant  Value=R2
  Constant3 : Constant  Value=R3
  Constant4 : Constant  Value=R4
  Gain : Gain  Gain=Rw
  Gain1 : Gain  Gain=1/Iwf
  Integrator : Integrator  InitialCondition=0.1
  MATLAB Function : MATLAB Function  TreatAsAtomicUnit=on
  MATLAB Function1 : MATLAB Function  TreatAsAtomicUnit=on
  Memory : Memory  InitialCondition=1
  One : Constant  OutDataTypeStr=Inherit: Inherit via back propagation
  Product : Product
  Scope : Scope  NumInputPorts=2
  Scope{2..4,8} (4 alike) : Scope
  Scope7 : Scope  NumInputPorts=2
  Sign : Signum
  Terminator : Terminator
  "Wr " : Outport  VectorParamsAs1DForOutWhenUnconnected=off
  RPM : Outport  Port=2  VectorParamsAs1DForOutWhenUnconnected=off
  shift : Outport  Port=3  VectorParamsAs1DForOutWhenUnconnected=off
  wires:
  One/1 -> Product/2
  Sign/1 -> Terminator/1
  Product/1 -> Add/3
  Add/1 -> Gain1/1, Scope8/1
  Tb_r/1 -> Product/1, Scope/2
  Constant1/1 -> MATLAB Function/4(R1)
  Constant2/1 -> MATLAB Function/3(R2)
  Constant3/1 -> MATLAB Function/2(R3)
  Constant4/1 -> MATLAB Function/1(R4)
  Memory/1 -> MATLAB Function1/1(u)
  MATLAB Function1/1(y) -> Add1/2
  Add1/1 -> MATLAB Function/6("shift "), shift/1
  Constant/1 -> Add1/1
  MATLAB Function/3(shift) -> Scope4/1, Memory/1
  MATLAB Function/1(y) -> "Wr "/1
  Integrator/1 -> MATLAB Function/5(u), Sign/1
  Ta/1 -> Add/1, Scope7/1  "Ta"
  Fxr/1 -> Gain/1
  Gain/1 -> Scope/1, Scope7/2, Add/2  "Fxr"
  Gain1/1 -> Scope3/1, Integrator/1
  MATLAB Function/2(RPM) -> RPM/1

== system Vehicle_Model_14DOF/Full vehicle 14 D.O.F /Vehicle Handling model 7D.O.F /Slip angle and beta /Slip angle front ==
  Xdot : Inport
  Delta : Inport  Port=2
  Ydot : Inport  Port=3
  Psidot : Inport  Port=4
  Add : Sum  Inputs=-+
  Add1 : Sum
  Atan : Trigonometry  Operator=atan
  Divide : Product  Inputs=*/
  Gain : Gain  Gain=a
  Scope{,1,3..5} (5 alike) : Scope
  Scope2 : Scope  NumInputPorts=2
  alpha_F : Outport  VectorParamsAs1DForOutWhenUnconnected=off
  wires:
  Gain/1 -> Add1/1
  Psidot/1 -> Gain/1, Scope3/1
  Xdot/1 -> Divide/2, Scope5/1
  Atan/1 -> Scope2/1, Add/2
  Divide/1 -> Scope/1, Atan/1
  Add1/1 -> Divide/1
  Ydot/1 -> Add1/2, Scope4/1
  Delta/1 -> Scope1/1, Scope2/2, Add/1
  Add/1 -> alpha_F/1

== system Vehicle_Model_14DOF/Full vehicle 14 D.O.F /Vehicle Handling model 7D.O.F /Slip angle and beta /Slip angle front1 ==
  Xdot : Inport
  Delta : Inport  Port=2
  Ydot : Inport  Port=3
  Psidot : Inport  Port=4
  Add : Sum  Inputs=-+
  Add1 : Sum
  Atan : Trigonometry  Operator=atan
  Divide : Product  Inputs=*/
  Gain : Gain  Gain=a
  Scope{,1,3..4} (4 alike) : Scope
  Scope2 : Scope  NumInputPorts=2
  alpha_F : Outport  VectorParamsAs1DForOutWhenUnconnected=off
  wires:
  Gain/1 -> Add1/1
  Psidot/1 -> Gain/1, Scope3/1
  Xdot/1 -> Divide/2
  Atan/1 -> Scope2/1, Add/2
  Divide/1 -> Scope/1, Atan/1
  Add1/1 -> Divide/1
  Ydot/1 -> Add1/2, Scope4/1
  Delta/1 -> Scope1/1, Scope2/2, Add/1
  Add/1 -> alpha_F/1

== system Vehicle_Model_14DOF/Full vehicle 14 D.O.F /Vehicle Handling model 7D.O.F /Slip angle and beta /Slip angle rear ==
  Xdot : Inport
  Ydot : Inport  Port=2
  Psidot : Inport  Port=3
  Add1 : Sum  Inputs=+-
  Atan : Trigonometry  Operator=atan
  Divide : Product  Inputs=*/
  Gain : Gain  Gain=b
  Scope : Scope
  Scope1 : Scope  NumInputPorts=2
  alpha_R : Outport  VectorParamsAs1DForOutWhenUnconnected=off
  wires:
  Gain/1 -> Scope1/1, Add1/2
  Psidot/1 -> Gain/1
  Xdot/1 -> Divide/2
  Divide/1 -> Atan/1
  Add1/1 -> Divide/1
  Ydot/1 -> Add1/1, Scope1/2
  Atan/1 -> alpha_R/1, Scope/1

== system Vehicle_Model_14DOF/Full vehicle 14 D.O.F /Vehicle Handling model 7D.O.F /Slip angle and beta /Slip angle rear1 ==
  Xdot : Inport
  Ydot : Inport  Port=2
  Psidot : Inport  Port=3
  Add1 : Sum  Inputs=+-
  Atan : Trigonometry  Operator=atan
  Divide : Product  Inputs=*/
  Gain : Gain  Gain=b
  Scope : Scope
  Scope1 : Scope  NumInputPorts=2
  alpha_R : Outport  VectorParamsAs1DForOutWhenUnconnected=off
  wires:
  Gain/1 -> Scope1/1, Add1/2
  Psidot/1 -> Gain/1
  Xdot/1 -> Divide/2
  Divide/1 -> Atan/1
  Add1/1 -> Divide/1
  Ydot/1 -> Add1/1, Scope1/2
  Atan/1 -> alpha_R/1, Scope/1

== system Vehicle_Model_14DOF/Full vehicle 14 D.O.F /Vehicle Handling model 7D.O.F /Slip ratio /Slip ratio Rear ==
  alpha R : Inport
  Xdot : Inport  Port=2
  y dot : Inport  Port=3
  psi dot : Inport  Port=4
  Wr : Inport  Port=5
  Add : Sum
  Add2 : Sum
  Constant : Constant
  Cos2 : Trigonometry  Operator=cos
  Divide : Product  Inputs=*/
  Gain : Gain  Gain=Rw
  Gain2 : Gain  Gain=b
  Multiply2 : Product
  Scope : Scope
  Scope1 : Scope
  Sqrt2 : Sqrt  SaturateOnIntegerOverflow=on
  Square4 : Math  Operator=square  SignedPower=on  SaturateOnIntegerOverflow=on
  Square5 : Math  Operator=square  SignedPower=on  SaturateOnIntegerOverflow=on
  Subtract : Sum  Inputs=-+
  Sum2 : Sum  Inputs=|+-
  sf : Outport  VectorParamsAs1DForOutWhenUnconnected=off
  wires:
  Xdot/1 -> Square4/1
  Cos2/1 -> Multiply2/1
  Square5/1 -> Add2/2
  Gain/1 -> Scope1/1, Divide/1
  Multiply2/1 -> Add/2  "wxr"
  Sum2/1 -> Square5/1
  Divide/1 -> Subtract/2
  Square4/1 -> Add2/1
  y dot/1 -> Sum2/1
  Add2/1 -> Sqrt2/1
  Wr/1 -> Gain/1
  Sqrt2/1 -> Multiply2/2  "Vtf"
  Gain2/1 -> Sum2/2
  psi dot/1 -> Gain2/1
  alpha R/1 -> Cos2/1
  Constant/1 -> Subtract/1
  Subtract/1 -> Scope/1, sf/1
  Add/1 -> Divide/2

== system Vehicle_Model_14DOF/Full vehicle 14 D.O.F /Vehicle Handling model 7D.O.F /Slip ratio /Slip ratio Rear1 ==
  alpha R : Inport
  Xdot : Inport  Port=2
  y dot : Inport  Port=3
  psi dot : Inport  Port=4
  Wr : Inport  Port=5
  Add : Sum
  Add2 : Sum
  Constant : Constant
  Cos2 : Trigonometry  Operator=cos
  Divide : Product  Inputs=*/
  Gain : Gain  Gain=Rw
  Gain2 : Gain  Gain=b
  Multiply2 : Product
  Scope : Scope
  Scope1 : Scope  NumInputPorts=2
  Sqrt2 : Sqrt  SaturateOnIntegerOverflow=on
  Square4 : Math  Operator=square  SignedPower=on  SaturateOnIntegerOverflow=on
  Square5 : Math  Operator=square  SignedPower=on  SaturateOnIntegerOverflow=on
  Subtract : Sum  Inputs=-+
  Sum2 : Sum  Inputs=|+-
  sf : Outport  VectorParamsAs1DForOutWhenUnconnected=off
  wires:
  Xdot/1 -> Square4/1
  Cos2/1 -> Multiply2/1
  Square5/1 -> Add2/2
  Gain/1 -> Scope1/1, Divide/1, Scope1/2
  Multiply2/1 -> Add/1  "wxr"
  Sum2/1 -> Square5/1
  Divide/1 -> Subtract/2
  Square4/1 -> Add2/1
  y dot/1 -> Sum2/1
  Add2/1 -> Sqrt2/1
  Wr/1 -> Gain/1
  Sqrt2/1 -> Multiply2/2  "Vtf"
  Gain2/1 -> Sum2/2
  psi dot/1 -> Gain2/1
  alpha R/1 -> Cos2/1
  Constant/1 -> Subtract/1
  Subtract/1 -> Scope/1, sf/1
  Add/1 -> Divide/2

== system Vehicle_Model_14DOF/Full vehicle 14 D.O.F /Vehicle Handling model 7D.O.F /Slip ratio /Slip ratio front ==
  Alpha F : Inport
  X dot : Inport  Port=2
  Y dot : Inport  Port=3
  psi dot : Inport  Port=4
  Wf : Inport  Port=5
  Add2 : Sum
  Constant : Constant
  Cos2 : Trigonometry  Operator=cos
  Divide : Product  Inputs=*/
  Gain : Gain  Gain=Rw
  Gain2 : Gain  Gain=a
  Multiply2 : Product
  Plus : Sum
  Scope : Scope
  Scope3 : Scope  NumInputPorts=2
  Sqrt2 : Sqrt  SaturateOnIntegerOverflow=on
  Square4 : Math  Operator=square  SignedPower=on  SaturateOnIntegerOverflow=on
  Square5 : Math  Operator=square  SignedPower=on  SaturateOnIntegerOverflow=on
  Subtract : Sum  Inputs=-+
  Sum2 : Sum  Inputs=|++
  sf : Outport  VectorParamsAs1DForOutWhenUnconnected=off
  wires:
  X dot/1 -> Square4/1
  Cos2/1 -> Multiply2/1
  Square5/1 -> Add2/2
  Gain/1 -> Divide/1, Scope3/1
  Multiply2/1 -> Plus/1  "wxr"
  Sum2/1 -> Square5/1
  Square4/1 -> Add2/1
  Y dot/1 -> Sum2/1
  Add2/1 -> Sqrt2/1
  Wf/1 -> Gain/1
  Sqrt2/1 -> Multiply2/2  "Vtf"
  Gain2/1 -> Sum2/2
  psi dot/1 -> Gain2/1
  Alpha F/1 -> Cos2/1
  Constant/1 -> Subtract/1
  Divide/1 -> Subtract/2
  Subtract/1 -> Scope/1, sf/1
  Plus/1 -> Scope3/2, Divide/2

== system Vehicle_Model_14DOF/Full vehicle 14 D.O.F /Vehicle Handling model 7D.O.F /Slip ratio /Slip ratio front1 ==
  Alpha F : Inport
  X dot : Inport  Port=2
  Y dot : Inport  Port=3
  psi dot : Inport  Port=4
  Wf : Inport  Port=5
  Add : Sum
  Add2 : Sum
  Constant : Constant
  Cos2 : Trigonometry  Operator=cos
  Divide : Product  Inputs=*/
  Gain : Gain  Gain=Rw
  Gain2 : Gain  Gain=a
  Multiply2 : Product
  Scope : Scope
  Scope1 : Scope
  Scope2 : Scope
  Scope3 : Scope  NumInputPorts=2
  Sqrt2 : Sqrt  SaturateOnIntegerOverflow=on
  Square4 : Math  Operator=square  SignedPower=on  SaturateOnIntegerOverflow=on
  Square5 : Math  Operator=square  SignedPower=on  SaturateOnIntegerOverflow=on
  Subtract : Sum  Inputs=-+
  Sum2 : Sum  Inputs=|++
  sf : Outport  VectorParamsAs1DForOutWhenUnconnected=off
  wires:
  X dot/1 -> Square4/1
  Cos2/1 -> Scope2/1, Multiply2/1
  Square5/1 -> Add2/2
  Gain/1 -> Divide/1, Scope3/1
  Multiply2/1 -> Add/1  "wxr"
  Sum2/1 -> Square5/1
  Square4/1 -> Add2/1
  Y dot/1 -> Sum2/1
  Add2/1 -> Sqrt2/1
  Wf/1 -> Gain/1
  Sqrt2/1 -> Multiply2/2  "Vtf"
  Gain2/1 -> Sum2/2
  psi dot/1 -> Gain2/1
  Alpha F/1 -> Scope1/1, Cos2/1
  Constant/1 -> Subtract/1
  Divide/1 -> Subtract/2
  Subtract/1 -> Scope/1, sf/1
  Add/1 -> Scope3/2, Divide/2

== system Vehicle_Model_14DOF/Full vehicle 14 D.O.F /Tiremodel/LCO width 6 psi 10/fy1/MZ ==
  Fz : Inport
  Slip angle : Inport  Port=2
  MATLAB Function : MATLAB Function  TreatAsAtomicUnit=on
  MZ : Outport  VectorParamsAs1DForOutWhenUnconnected=off
  wires:
  Fz/1 -> MATLAB Function/1(ffz)
  Slip angle/1 -> MATLAB Function/2(xx)
  MATLAB Function/1(Fx) -> MZ/1

== system Vehicle_Model_14DOF/Full vehicle 14 D.O.F /Tiremodel/LCO width 6 psi 14/fy1/MZ ==
  Fz : Inport
  Slip angle : Inport  Port=2
  MATLAB Function : MATLAB Function  TreatAsAtomicUnit=on
  MZ : Outport  VectorParamsAs1DForOutWhenUnconnected=off
  wires:
  Fz/1 -> MATLAB Function/1(ffz)
  Slip angle/1 -> MATLAB Function/2(xx)
  MATLAB Function/1(Fx) -> MZ/1

== system Vehicle_Model_14DOF/Full vehicle 14 D.O.F /Tiremodel/R25b width 6 psi 10/fy1/MZ ==
  Fz : Inport
  Slip angle : Inport  Port=2
  MATLAB Function : MATLAB Function  TreatAsAtomicUnit=on
  MZ : Outport  VectorParamsAs1DForOutWhenUnconnected=off
  wires:
  Fz/1 -> MATLAB Function/1(ffz)
  Slip angle/1 -> MATLAB Function/2(xx)
  MATLAB Function/1(Fx) -> MZ/1

== system Vehicle_Model_14DOF/Full vehicle 14 D.O.F /Tiremodel/R25b width 6 psi 14/fy1/MZ ==
  Fz : Inport
  Slip angle : Inport  Port=2
  MATLAB Function : MATLAB Function  TreatAsAtomicUnit=on
  MZ : Outport  VectorParamsAs1DForOutWhenUnconnected=off
  wires:
  Fz/1 -> MATLAB Function/1(ffz)
  Slip angle/1 -> MATLAB Function/2(xx)
  MATLAB Function/1(Fx) -> MZ/1

== system Vehicle_Model_14DOF/Full vehicle 14 D.O.F /Tiremodel/R25b width 7 psi 10/MZ/MZ ==
  Fz : Inport
  Slip angle : Inport  Port=2
  MATLAB Function : MATLAB Function  TreatAsAtomicUnit=on
  MZ : Outport  VectorParamsAs1DForOutWhenUnconnected=off
  wires:
  Fz/1 -> MATLAB Function/1(ffz)
  Slip angle/1 -> MATLAB Function/2(xx)
  MATLAB Function/1(Fx) -> MZ/1

== system Vehicle_Model_14DOF/Full vehicle 14 D.O.F /Tiremodel/R25b width 7 psi 14/fy1/MZ ==
  Fz : Inport
  Slip angle : Inport  Port=2
  MATLAB Function : MATLAB Function  TreatAsAtomicUnit=on
  MZ : Outport  VectorParamsAs1DForOutWhenUnconnected=off
  wires:
  Fz/1 -> MATLAB Function/1(ffz)
  Slip angle/1 -> MATLAB Function/2(xx)
  MATLAB Function/1(Fx) -> MZ/1

== system Vehicle_Model_14DOF/Full vehicle 14 D.O.F /Tiremodel/Tire front left/fy1/MZ ==
  Fz : Inport
  Slip angle : Inport  Port=2
  MATLAB Function : MATLAB Function  TreatAsAtomicUnit=on
  MZ : Outport  VectorParamsAs1DForOutWhenUnconnected=off
  wires:
  Fz/1 -> MATLAB Function/1(ffz)
  Slip angle/1 -> MATLAB Function/2(xx)
  MATLAB Function/1(Fx) -> MZ/1

== system Vehicle_Model_14DOF/Full vehicle 14 D.O.F /Tiremodel/Tire front right/fy1/MZ ==
  Fz : Inport
  Slip angle : Inport  Port=2
  MATLAB Function : MATLAB Function  TreatAsAtomicUnit=on
  MZ : Outport  VectorParamsAs1DForOutWhenUnconnected=off
  wires:
  MATLAB Function/1(Fx) -> MZ/1
  Slip angle/1 -> MATLAB Function/2(xx)
  Fz/1 -> MATLAB Function/1(ffz)

== system Vehicle_Model_14DOF/Full vehicle 14 D.O.F /Tiremodel/Tire rear Right/fy1/MZ ==
  Fz : Inport
  Slip angle : Inport  Port=2
  MATLAB Function : MATLAB Function  TreatAsAtomicUnit=on
  MZ : Outport  VectorParamsAs1DForOutWhenUnconnected=off
  wires:
  Fz/1 -> MATLAB Function/1(ffz)
  Slip angle/1 -> MATLAB Function/2(xx)
  MATLAB Function/1(Fx) -> MZ/1

== system Vehicle_Model_14DOF/Full vehicle 14 D.O.F /Tiremodel/Tire rear left/fy1/MZ ==
  Fz : Inport
  Slip angle : Inport  Port=2
  MATLAB Function : MATLAB Function  TreatAsAtomicUnit=on
  MZ : Outport  VectorParamsAs1DForOutWhenUnconnected=off
  wires:
  MATLAB Function/1(Fx) -> MZ/1
  Slip angle/1 -> MATLAB Function/2(xx)
  Fz/1 -> MATLAB Function/1(ffz)

== matlab function Vehicle_Model_14DOF/Full vehicle 14 D.O.F /Tiremodel/Tire rear Right/fy1/MZ/MATLAB Function ==
  data: ffz input; Fx output; xx input
function Fx = fcn(ffz,xx)

%xx is the slip ratio -- expressed as fraction
D = -2.0312
C = -0.0268
B = 1.0528
E = 1.1437


Fx = D.* ffz .*sin(C.* atan((B.*(xx))- E*(B.* (xx)- atan(B.*(xx))))) ;

== matlab function Vehicle_Model_14DOF/Full vehicle 14 D.O.F /Subsystem/MATLAB Function ==
  data: Ackerman input; Ackerman_inner output; a input; b input; Wf input; Percent input
function Ackerman_inner= fcn(Ackerman,a,b,Wf,Percent)

Ackerman_inner = 180/pi.*atan((a+b)/((a+b)./(tan(pi.*Ackerman/180))-Wf)).*Percent;

== matlab function Vehicle_Model_14DOF/MATLAB Function ==
  data: Ay input; gs output; Ax input
function gs = fcn(Ay,Ax)

gs = sqrt((Ax.^2+Ay.^2));

== matlab function Vehicle_Model_14DOF/Full vehicle 14 D.O.F /Vehicle Handling model 7D.O.F /Powertrain /MATLAB Function2 ==
  data: T input; Fx input; RPM input; m output; Rw input
function m = fcn(T, Fx, RPM, Rw)
if (RPM > 15100)
    m = Fx *Rw;
else
    m=T;
end
end

== matlab function Vehicle_Model_14DOF/Full vehicle 14 D.O.F /Vehicle Handling model 7D.O.F /Powertrain /MATLAB Function3 ==
  data: T input; Fx input; RPM input; m output; Rw input
function m = fcn(T, Fx, RPM, Rw)
if (RPM > 15100)
    m = Fx * Rw;
else
    m= T;
end
end

== matlab function Vehicle_Model_14DOF/Full vehicle 14 D.O.F /Vehicle Handling model 7D.O.F /Powertrain /MATLAB Function ==
  data: R4 input; R3 input; R2 input; t input; R1 input; m output; shift input
function m = fcn(R4, R3, R2, t, R1, shift)
if (shift ==1)
    m= t *R1
elseif (shift ==2)
    m= t * R2
elseif (shift ==3)
     m= t * R3
elseif (shift ==4)
      m= t * R4
else
    m=1
end

== matlab function Vehicle_Model_14DOF/Full vehicle 14 D.O.F /Vehicle Handling model 7D.O.F /Powertrain /rear wheel spin/MATLAB Function ==
  data: R4 input; R3 input; R2 input; R1 input; u input; y output; RPM output; shift output; shift input
function [y, RPM, shift]= fcn(R4, R3, R2, R1, u, shift)
ratio =[R1 R2 R3 R4]
RPM = 10*u * ratio(shift)
low = [1, 10898, 12475,13119]
if RPM >= 15000 && shift <4 
shift = shift + 1
end

if (shift >1)
if (RPM < (15000* ratio (shift) / ratio(shift-1)))
    shift = shift -1
end
end
y = u
RPM =RPM
shift = shift;

== matlab function Vehicle_Model_14DOF/Full vehicle 14 D.O.F /Vehicle Handling model 7D.O.F /Powertrain /rear wheel spin/MATLAB Function1 ==
  data: u input; y output
function y = fcn(u)

if (u ==1)
    y=0  
else    y=u-1 
end

== matlab function Vehicle_Model_14DOF/Full vehicle 14 D.O.F /Vehicle Handling model 7D.O.F /Powertrain /MATLAB Function1 ==
  data: R4 input; R3 input; R2 input; t input; R1 input; m output; shifts input
function m = fcn(R4, R3, R2, t, R1, shifts)
if (shifts ==1)
    m= t *R1
elseif (shifts ==2)
    m= t * R2
elseif (shifts ==3)
     m= t * R3
elseif (shifts ==4)
      m= t * R4
else
    m=1
end

== matlab function Vehicle_Model_14DOF/Full vehicle 14 D.O.F /Vehicle Handling model 7D.O.F /Powertrain /rear wheel spin1/MATLAB Function ==
  data: R4 input; R3 input; R2 input; R1 input; u input; y output; RPM output; shift output; shift input
function [y, RPM, shift]= fcn(R4, R3, R2, R1, u, shift)
ratio =[R1 R2 R3 R4]
RPM = 10*u * ratio(shift)
low = [1, 10898, 12475,13119]
if RPM >= 15000 && shift <4 
shift = shift + 1
end

if (shift >1)
if (RPM < (15000* ratio (shift) / ratio(shift-1)))
    shift = shift -1
end
end
y = u
RPM =RPM
shift = shift;

== matlab function Vehicle_Model_14DOF/Full vehicle 14 D.O.F /Vehicle Handling model 7D.O.F /Powertrain /rear wheel spin1/MATLAB Function1 ==
  data: u input; y output
function y = fcn(u)

if (u ==1)
    y=0  
else    y=u-1 
end

== matlab function Vehicle_Model_14DOF/Full vehicle 14 D.O.F /Vehicle Handling model 7D.O.F /Longtudinal axis D.O.F /centriptal Accelration deduction  ==
  data: Vx_dot input; Ax output; Vy input; Yr input
function Ax = fcn(Vx_dot,Vy,Yr)

Ax = Vx_dot+(Vy.*Yr);

== matlab function Vehicle_Model_14DOF/Full vehicle 14 D.O.F /Vehicle Handling model 7D.O.F /Lateral Axis D.o.f /Centripital force deduction ay  ==
  data: Vy_dot input; ay output; Vx input; Yr input
function ay = fcn(Vy_dot,Vx,Yr)

ay = Vy_dot-(Vx.*Yr);
